simulink model "UDPPlayground"  (R2024b)
settings: Solver=FixedStepAuto  StartTime=0.0  StopTime=inf  RelTol=1e-3  EnableMultiTasking=on
values from neighbouring files (symbols this model uses):
  tx_id_sensor2 = 2    [UDPPlayground_Vars.m]
  tx_id_sensor3 = 3    [UDPPlayground_Vars.m]
undefined symbols (not defined in the file or in its folder): portbindings
libraries: bbblueCommlib x17, simulink_extras x2, sharedtransform x1
settings Model: ExtModeTrigDuration=100  Creator=Henrik  LastModifiedBy=Henrik
settings SolverCC: PositivePriorityOrder=on  AutoInsertRateTranBlk=on
settings OptimizationCC: DefaultParameterBehavior=Inlined  EnhancedBackFolding=on  PassReuseOutputArgsAs=Individual arguments  ZeroExternalMemoryAtStartup=off  ZeroInternalMemoryAtStartup=off  MaxStackSize=64  OptimizeBlockOrder=speed  DifferentSizesBufferReuse=on  OptimizationCustomize=off  EfficientTunableParamExpr=on
settings DebuggingCC: ParameterTunabilityLossMsg=error
settings HardwareCC: ProdBitPerPointer=32  ProdBitPerSizeT=32  ProdBitPerPtrDiffT=32  ProdLargestAtomicInteger=Long  ProdLargestAtomicFloat=Double  ProdWordSize=32  ProdHWDeviceType=ARM Compatible->ARM Cortex-A (32-bit)  UseEmbeddedCoderFeatures=off
settings SFSimCC: MATLABDynamicMemAlloc=off
settings RTWCC: Description=Embedded Coder  SystemTargetFile=ert.tlc  HardwareBoard=BeagleBone Blue  TLCOptions="-aInlineSetEventsForThisBaseRateFcn=TLC_FALSE -aSuppressMultiTaskScheduler=TLC_FALSE  -aRateBasedStepFcn=0"  TemplateMakefile=ert_default_tmf  Toolchain=GNU GCC BeagleBone Blue
settings CodeAppCC: ForceParamTrailComments=on  IgnoreCustomStorageClasses=off  OperatorAnnotations=on  SimulinkDataObjDesc=on  SFDataObjDesc=on  InsertBlockDesc=on
settings ERTTargetCC: SupportNonInlinedSFcns=on  SupportVariableSizeSignals=on

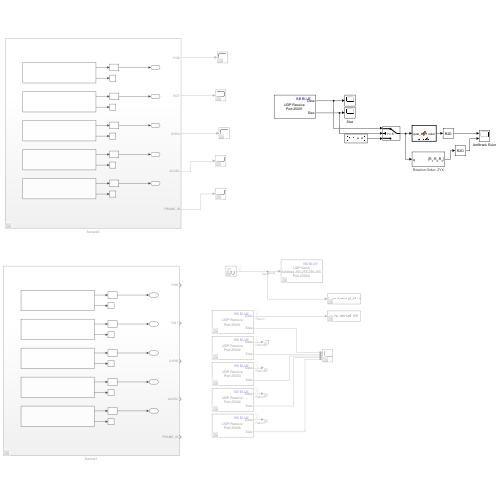
[thumbnail: Simulink's stored preview of the top-level diagram]
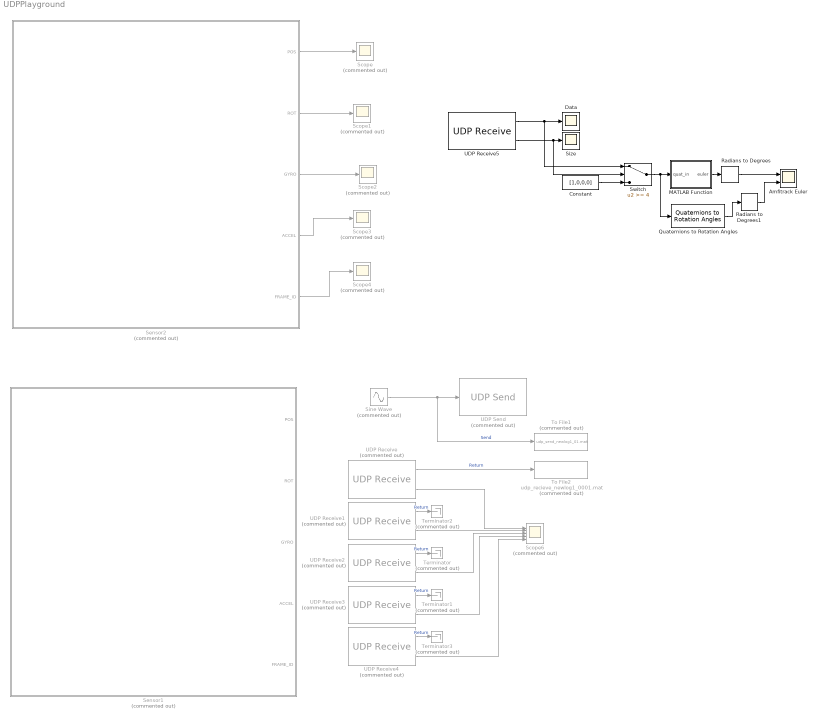
== system UDPPlayground ==
  Amfitrack Euler : Scope  NumInputPorts=2
  Constant : Constant  Value=[1,0,0,0]
  Data : Scope
  MATLAB Function : MATLAB Function  TreatAsAtomicUnit=on
  Quaternions to Rotation Angles : sharedtransform/Quaternions to Rotation Angles  rotationOrder=ZYX  aMode=aMode
  Radians to Degrees : simulink_extras/Transformations/Radians to Degrees
  Radians to Degrees1 : simulink_extras/Transformations/Radians to Degrees
  Scope{,1..4} (5 alike) : Scope  Commented=on
  Scope6 : Scope  Commented=on  NumInputPorts=5
  Sensor1 : Subsystem  Commented=on
  Sensor2 : Subsystem  Commented=on
  Sine Wave : Sin  Commented=on  Amplitude=50  SampleTime=0.1
  Size : Scope
  Switch : Switch  Threshold=4  SaturateOnIntegerOverflow=off  InputSameDT=off
  Terminator{,1..3} (4 alike) : Terminator  Commented=on
  To File1 : ToFile  Commented=on  Filename=udp_send_newlog1_01.mat
  To File2 : ToFile  Commented=on  Filename=udp_recieve_newlog1_0001.mat
  UDP Receive : bbblueCommlib/UDP Receive  Commented=on  localURL='0.0.0.0'  localPort=25001  remoteURL='0.0.0.0'  remotePort=-1  recvBufferSize=8192  signalDatatype=double  dims=255  isVarSize=off  showBlockingTime=off  blockingTime=0  sampletime=0.001  blockPlatform=BB BLUE
  UDP Receive1 : bbblueCommlib/UDP Receive  Commented=on  localURL='0.0.0.0'  localPort=25002  remoteURL='0.0.0.0'  remotePort=-1  recvBufferSize=8192  signalDatatype=double  dims=255  isVarSize=off  showBlockingTime=off  blockingTime=0  sampletime=0.001  blockPlatform=BB BLUE
  UDP Receive2 : bbblueCommlib/UDP Receive  Commented=on  localURL='0.0.0.0'  localPort=25003  remoteURL='0.0.0.0'  remotePort=-1  recvBufferSize=8192  signalDatatype=double  dims=255  isVarSize=off  showBlockingTime=off  blockingTime=0  sampletime=0.001  blockPlatform=BB BLUE
  UDP Receive3 : bbblueCommlib/UDP Receive  Commented=on  localURL='0.0.0.0'  localPort=25004  remoteURL='0.0.0.0'  remotePort=-1  recvBufferSize=8192  signalDatatype=double  dims=255  isVarSize=off  showBlockingTime=off  blockingTime=0  sampletime=0.001  blockPlatform=BB BLUE
  UDP Receive4 : bbblueCommlib/UDP Receive  Commented=on  localURL='0.0.0.0'  localPort=25005  remoteURL='0.0.0.0'  remotePort=-1  recvBufferSize=8192  signalDatatype=double  dims=255  isVarSize=off  showBlockingTime=off  blockingTime=0  sampletime=0.001  blockPlatform=BB BLUE
  UDP Receive5 : bbblueCommlib/UDP Receive  localURL='0.0.0.0'  localPort=25001  remoteURL='0.0.0.0'  remotePort=-1  recvBufferSize=8192  signalDatatype=double  dims=4  isVarSize=off  showBlockingTime=off  blockingTime=0  sampletime=0.01  blockPlatform=BB BLUE
  UDP Send : bbblueCommlib/UDP Send  Commented=on  remoteURL='255.255.255.255'  remotePort=25000  localURL='0.0.0.0'  localPortSource=Automatically determine  localPort=2048  sendBufferSize=8192  sampletime=-1  blockPlatform=BB BLUE  separateLengthPort=0
  wires:
  Sensor2/1(POS) -> Scope/1
  Sensor2/2(ROT) -> Scope1/1
  Sensor2/3(GYRO) -> Scope2/1
  Sensor2/4(ACCEL) -> Scope3/1
  Sensor2/5(FRAME_ID) -> Scope4/1
  Sine Wave/1 -> To File1/1, UDP Send/1  "Send"
  UDP Receive/1 -> To File2/1  "Return"
  UDP Receive/2 -> Scope6/1
  UDP Receive1/2 -> Scope6/2
  UDP Receive2/1 -> Terminator/1  "Return"
  UDP Receive1/1 -> Terminator2/1  "Return"
  UDP Receive3/1 -> Terminator1/1  "Return"
  UDP Receive4/1 -> Terminator3/1  "Return"
  UDP Receive4/2 -> Scope6/5
  UDP Receive3/2 -> Scope6/4
  UDP Receive2/2 -> Scope6/3
  UDP Receive5/1 -> Switch/1, Data/1
  UDP Receive5/2 -> Switch/2, Size/1
  MATLAB Function/1(euler) -> Radians to Degrees/1
  Switch/1 -> Quaternions to Rotation Angles/1, MATLAB Function/1(quat_in)
  Constant/1 -> Switch/3
  Radians to Degrees/1 -> Amfitrack Euler/1
  Quaternions to Rotation Angles/1 -> Radians to Degrees1/1
  Radians to Degrees1/1 -> Amfitrack Euler/2

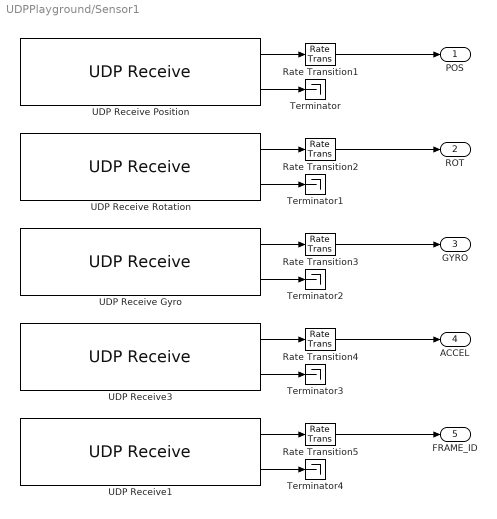
== system UDPPlayground/Sensor1 ==
  Rate Transition{1..5} (5 alike) : RateTransition  OutPortSampleTime=0.02
  Terminator{,1..4} (5 alike) : Terminator
  UDP Receive Gyro : bbblueCommlib/UDP Receive  localURL='0.0.0.0'  localPort=2000 + 100 * tx_id_sensor3 + portbindings.GYRO  remoteURL='0.0.0.0'  remotePort=-1  recvBufferSize=8192  signalDatatype=uint8  dims=255  isVarSize=off  showBlockingTime=off  blockingTime=0  sampletime=0.1  blockPlatform=BB BLUE
  UDP Receive Position : bbblueCommlib/UDP Receive  localURL='0.0.0.0'  localPort=2000 + 100 * tx_id_sensor3 + portbindings.POS  remoteURL='0.0.0.0'  remotePort=-1  recvBufferSize=8192  signalDatatype=uint8  dims=255  isVarSize=off  showBlockingTime=off  blockingTime=0  sampletime=0.1  blockPlatform=BB BLUE
  UDP Receive Rotation : bbblueCommlib/UDP Receive  localURL='0.0.0.0'  localPort=2000 + 100 * tx_id_sensor3 + portbindings.ROT  remoteURL='0.0.0.0'  remotePort=-1  recvBufferSize=8192  signalDatatype=uint8  dims=255  isVarSize=off  showBlockingTime=off  blockingTime=0  sampletime=0.1  blockPlatform=BB BLUE
  UDP Receive1 : bbblueCommlib/UDP Receive  localURL='0.0.0.0'  localPort=2000 + 100 * tx_id_sensor3 + portbindings.FRAME_ID  remoteURL='0.0.0.0'  remotePort=-1  recvBufferSize=8192  signalDatatype=uint8  dims=255  isVarSize=off  showBlockingTime=off  blockingTime=0  sampletime=0.1  blockPlatform=BB BLUE
  UDP Receive3 : bbblueCommlib/UDP Receive  localURL='0.0.0.0'  localPort=2000 + 100 * tx_id_sensor3 + portbindings.ACCEL  remoteURL='0.0.0.0'  remotePort=-1  recvBufferSize=8192  signalDatatype=uint8  dims=255  isVarSize=off  showBlockingTime=off  blockingTime=0  sampletime=0.1  blockPlatform=BB BLUE
  POS : Outport
  ROT : Outport  Port=2
  GYRO : Outport  Port=3
  ACCEL : Outport  Port=4
  FRAME_ID : Outport  Port=5
  wires:
  UDP Receive Rotation/1 -> Rate Transition2/1
  UDP Receive3/2 -> Terminator3/1
  UDP Receive Position/1 -> Rate Transition1/1
  UDP Receive Gyro/1 -> Rate Transition3/1
  UDP Receive Rotation/2 -> Terminator1/1
  UDP Receive Position/2 -> Terminator/1
  UDP Receive Gyro/2 -> Terminator2/1
  UDP Receive3/1 -> Rate Transition4/1
  UDP Receive1/2 -> Terminator4/1
  Rate Transition4/1 -> ACCEL/1
  UDP Receive1/1 -> Rate Transition5/1
  Rate Transition1/1 -> POS/1
  Rate Transition3/1 -> GYRO/1
  Rate Transition2/1 -> ROT/1
  Rate Transition5/1 -> FRAME_ID/1

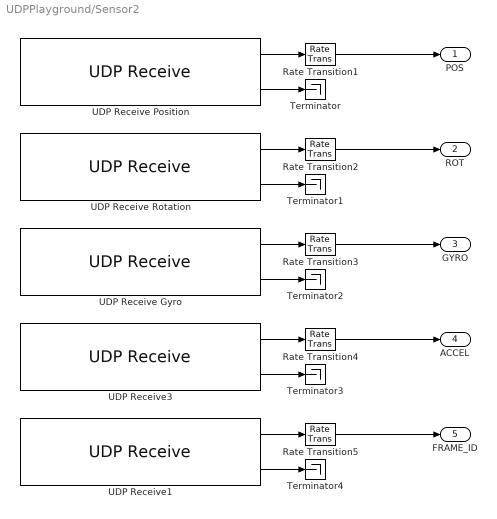
== system UDPPlayground/Sensor2 ==
  Rate Transition{1..5} (5 alike) : RateTransition  OutPortSampleTime=0.02
  Terminator{,1..4} (5 alike) : Terminator
  UDP Receive Gyro : bbblueCommlib/UDP Receive  localURL='0.0.0.0'  localPort=2000 + 100 * tx_id_sensor2 + portbindings.GYRO  remoteURL='0.0.0.0'  remotePort=-1  recvBufferSize=8192  signalDatatype=uint8  dims=255  isVarSize=off  showBlockingTime=off  blockingTime=0  sampletime=0.1  blockPlatform=BB BLUE
  UDP Receive Position : bbblueCommlib/UDP Receive  localURL='0.0.0.0'  localPort=2000 + 100 * tx_id_sensor2 + portbindings.POS  remoteURL='0.0.0.0'  remotePort=-1  recvBufferSize=8192  signalDatatype=uint8  dims=255  isVarSize=off  showBlockingTime=off  blockingTime=0  sampletime=0.1  blockPlatform=BB BLUE
  UDP Receive Rotation : bbblueCommlib/UDP Receive  localURL='0.0.0.0'  localPort=2000 + 100 * tx_id_sensor2 + portbindings.ROT  remoteURL='0.0.0.0'  remotePort=-1  recvBufferSize=8192  signalDatatype=uint8  dims=255  isVarSize=off  showBlockingTime=off  blockingTime=0  sampletime=0.1  blockPlatform=BB BLUE
  UDP Receive1 : bbblueCommlib/UDP Receive  localURL='0.0.0.0'  localPort=2000 + 100 * tx_id_sensor2 + portbindings.FRAME_ID  remoteURL='0.0.0.0'  remotePort=-1  recvBufferSize=8192  signalDatatype=uint8  dims=255  isVarSize=off  showBlockingTime=off  blockingTime=0  sampletime=0.1  blockPlatform=BB BLUE
  UDP Receive3 : bbblueCommlib/UDP Receive  localURL='0.0.0.0'  localPort=2000 + 100 * tx_id_sensor2 + portbindings.ACCEL  remoteURL='0.0.0.0'  remotePort=-1  recvBufferSize=8192  signalDatatype=uint8  dims=255  isVarSize=off  showBlockingTime=off  blockingTime=0  sampletime=0.1  blockPlatform=BB BLUE
  POS : Outport
  ROT : Outport  Port=2
  GYRO : Outport  Port=3
  ACCEL : Outport  Port=4
  FRAME_ID : Outport  Port=5
  wires:
  UDP Receive Rotation/1 -> Rate Transition2/1
  UDP Receive3/2 -> Terminator3/1
  UDP Receive Position/1 -> Rate Transition1/1
  UDP Receive Gyro/1 -> Rate Transition3/1
  UDP Receive Rotation/2 -> Terminator1/1
  UDP Receive Position/2 -> Terminator/1
  UDP Receive Gyro/2 -> Terminator2/1
  UDP Receive3/1 -> Rate Transition4/1
  UDP Receive1/2 -> Terminator4/1
  Rate Transition4/1 -> ACCEL/1
  UDP Receive1/1 -> Rate Transition5/1
  Rate Transition1/1 -> POS/1
  Rate Transition3/1 -> GYRO/1
  Rate Transition2/1 -> ROT/1
  Rate Transition5/1 -> FRAME_ID/1

== matlab function UDPPlayground/MATLAB Function ==
  data: quat_in input; euler output
function euler = to_euler(quat_in)

q0 = quat_in(1);
q1 = quat_in(2);
q2 = quat_in(3);
q3 = quat_in(4);

roll = atan((2 * (q0*q1 + q2*q3))/(1 - 2*(q1^2 + q2^2)));
pitch = asin(2 * (q0*q2 - q1*q3));
yaw = atan2((2 * (q0*q3 + q1*q2)),(1 - 2*(q2^2 + q3^2)));

euler = [roll; pitch; yaw];
